simulink model "MPPT"  (R2022a)
settings: Solver=VariableStepAuto  StartTime=0.0  StopTime=0.01  RelTol=1e-3
libraries: spsSeriesRLCBranchLib x4, spsCurrentMeasurementLib x2, spsVoltageMeasurementLib x2, spsDiodeLib x1, spsIGBTDiodeLib x1, spsPVArrayLib x1, spsPWMGeneratorDCDCLib x1, spspowerguiLib x1
settings Model: Creator=nikke  LastModifiedBy=nikke

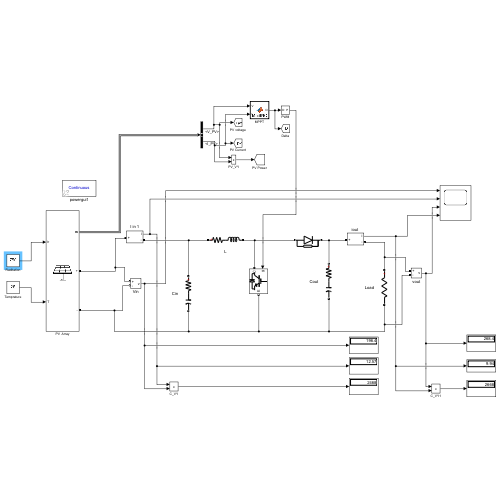
[thumbnail: Simulink's stored preview of the top-level diagram]
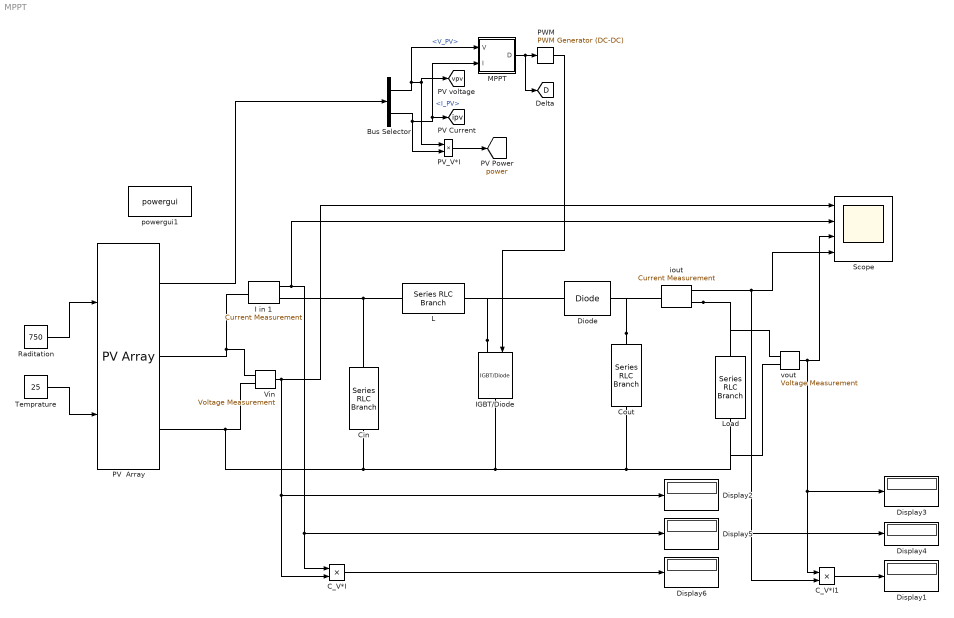
== system MPPT ==
  Bus Selector : BusSelector  OutputSignals=V_PV,I_PV
  C_V*I : Product
  C_V*I1 : Product
  Cin : spsSeriesRLCBranchLib/Series RLC Branch  LConnTagsString=__new0  RConnTagsString=__new0  BranchType=RC  Resistance=1e-4  Inductance=1e-3  SetiL0=off  InitialCurrent=0  Capacitance=100e-6  Setx0=off  InitialVoltage=0  Measurements=None
  Cout : spsSeriesRLCBranchLib/Series RLC Branch  LConnTagsString=__new0  RConnTagsString=__new0  BranchType=RC  Resistance=0.0001  Inductance=1e-3  SetiL0=off  InitialCurrent=0  Capacitance=100e-6  Setx0=off  InitialVoltage=0  Measurements=None
  Diode : spsDiodeLib/Diode  Ron=0.001  Lon=0  Vf=0.8  IC=0  UseSnubber=off  Rs=500  Cs=250e-9  Measurements=off
  Display{1..6} (6 alike) : Display
  I in 1 : spsCurrentMeasurementLib/Current Measurement  PhasorSimulation=off  OutputType=Complex  PSBequivalent=0
  IGBT/Diode : spsIGBTDiodeLib/IGBT//Diode  Ron=1e-3  Rs=1e5  Cs=inf  Measurements=off
  L : spsSeriesRLCBranchLib/Series RLC Branch  LConnTagsString=__new0  RConnTagsString=__new0  BranchType=RL  Resistance=0.1  Inductance=2e-3  SetiL0=off  InitialCurrent=0  Capacitance=100e-6  Setx0=off  InitialVoltage=0  Measurements=None
  Load : spsSeriesRLCBranchLib/Series RLC Branch  LConnTagsString=__new0  RConnTagsString=__new0  BranchType=R  Resistance=27  Inductance=1e-3  SetiL0=off  InitialCurrent=0  Capacitance=100e-6  Setx0=off  InitialVoltage=0  Measurements=None
  MPPT : MATLAB Function  TreatAsAtomicUnit=on
  PV  Array : spsPVArrayLib/PV Array  Npar=2  Nser=12  PlotType=array @ 1000 W/m2 & specified temperatures  S_vec="[ 1000  500  100 ]"  Temp_C_vec="[ 45 25  ]"  ModuleName=Tata Power Solar Systems TP140SBZ  PlotWhenSelected=off  Pm=139.6944  Ncell=36  Voc=22.25  Isc=8.66  Vm=17.44  Im=8.01  beta_Voc_pc=-0.33  alpha_Isc_pc=0.063799  beta_Voc=-0.073425  alpha_Isc=0.005525  IL=8.6872  I0=9.8965e-11  nI=0.95579  Rsh=88.7762  Rs=0.27837  RobustModel=off  RobustCellTemperature=313.3991  BAL=on  Tc=1e-6  Tfilter=5e-5
  PV_V*I : Product
  PWM : spsPWMGeneratorDCDCLib/PWM Generator (DC-DC)  Fsw=5000  Ts=5e-6
  Raditation : Constant  Value=750
  Scope : Scope  NumInputPorts=4
  Temprature : Constant  Value=25
  "Vin " : spsVoltageMeasurementLib/Voltage Measurement  PhasorSimulation=off  OutputType=Complex  PSBequivalent=0
  "iout " : spsCurrentMeasurementLib/Current Measurement  PhasorSimulation=off  OutputType=Complex  PSBequivalent=0
  powergui1 : spspowerguiLib/powergui  Priority=1  SimulationMode=Continuous  SampleTime=50e-6  frequency=60  Iterations=50  frequencyindice=0  Pbase=100e6  ErrMax=1e-4  UnitsV=kV  UnitsW=MW  buscounter=0  FunctionMessages=off  echomessages=off  EnableUseOfTLC=off  CurrentSourceSwitches=off  DisableSnubberDevices=off  DisableRonSwitches=off  DisableVfSwitches=off  DisplayEquations=off  AutomaticDiscreteSolvers=off  SolverType=Tustin/Backward Euler (TBE)  Interpol=off  ExternalGateDelay=off  methode=off  Ts=100  x0status=blocks  SPID=on  SwTol=0  HookPort=off  NonlinearTolerance=1e-4  nMaxIteration=100  ContinueOnMaxIteration=off  RestoreLinks=warning  ResistiveCurrentMeasurement=off  Frange=[0:2:500]  Ylog=off  Xlog=on  ShowGrid=off  save=off  variable=ZData  structure=0  ZoomFFT=off  StartTime=0.0  cycles=1  DisplayStyle=1  fundamental=60  FreqAxis=off  MaxFrequency=1000  frequencyindicesteady=1  RmsSteady=1  display=off
  "vout " : spsVoltageMeasurementLib/Voltage Measurement  PhasorSimulation=off  OutputType=Complex  PSBequivalent=0
  tag scope: D=global, ipv=global, power=global, vpv=global
  wires:
  Bus Selector/2 -> MPPT/2(I), [ipv], PV_V*I/2  "<I_PV>"
  PV_V*I/1 -> [power]
  Bus Selector/1 -> [vpv], PV_V*I/1, MPPT/1(V)  "<V_PV>"
  PV  Array/1 -> Bus Selector/1
  PWM/1 -> IGBT/Diode/1
  MPPT/1(D) -> PWM/1, [D]
  "iout "/1 -> Display4/1, C_V*I1/2, Scope/4
  "vout "/1 -> Display3/1, C_V*I1/1, Scope/3
  Temprature/1 -> PV  Array/2
  C_V*I/1 -> Display6/1
  I in 1/1 -> Display5/1, C_V*I/1, Scope/2
  C_V*I1/1 -> Display1/1
  "Vin "/1 -> C_V*I/2, Display2/1, Scope/1
  Raditation/1 -> PV  Array/1
  connections:
  IGBT/Diode/RConn1 -- Load/RConn1 -- "vout "/LConn2 -- Cout/RConn1 -- "Vin "/LConn2 -- PV  Array/RConn2 -- Cin/RConn1
  IGBT/Diode/LConn1 -- L/RConn1 -- Diode/LConn1
  I in 1/RConn1 -- Cin/LConn1 -- L/LConn1
  "iout "/RConn1 -- Load/LConn1 -- "vout "/LConn1
  Cout/LConn1 -- Diode/RConn1 -- "iout "/LConn1
  "Vin "/LConn1 -- I in 1/LConn1 -- PV  Array/RConn1

== matlab function MPPT/MPPT ==
  settings: updateMethod=DISCRETE
  data: V input; D output; I input
% author : Saad MOTAHHIR
% f=1000hz
function D  = ModINC(V, I)


Dinit = 0.6;  %Initial value for D output
Dmax = 0.65;   %Maximum value for D
Dmin = 0.1;   %Minimum value for D
deltaD = 0.0007; %Increment value used to increase/decrease the duty cycle D

  
persistent Vold Pold Dold Iold M;

dataType = 'double';

if isempty(Vold)
    Vold=0;
    Pold=0;
    Iold=0;
    Dold=Dinit;
    M=1;
end
P= V*I;
dV= V - Vold;
dP= P - Pold;
dI= I - Iold;
M=abs(dP);

if M < 0.005
    D=Dold;
else
    if dV == 0
        if dI == 0
            D=Dold;
        elseif dI>0
            D=Dold - (M*deltaD);
        else 
            D=Dold + (M*deltaD);
        end    
    else
        if dI/dV == -I/V
            D=Dold;
        elseif dI/dV>-I/V    
           D=Dold - (M*deltaD);
        else
           D=Dold + (M*deltaD);  
        end  
    end    
end

if D >= Dmax | D<= Dmin
    D=Dold;
end

Dold=D;
Vold=V;
Pold=P;
Iold=I;
